simulink model "raman_updated"  (R2024b)
settings: Solver=VariableStepAuto  StartTime=0.0  StopTime=10.0  RelTol=1e-3
values from neighbouring files (symbols this model uses):
  alpha_AS_dB_km = 0.40    (= 0.4)    [Inverter_new.m]    (also in init_pv_inverter.m = 0.26)
  alpha_p_dB_km = 0.20    (= 0.2)    [Inverter_new.m]    (also in init_pv_inverter.m)
  alpha_S_dB_km = 0.20    (= 0.2)    [Inverter_new.m]    (also in init_pv_inverter.m = 0.24)
  B_rx = 1e9    (= 1000000000)    [Inverter_new.m]    (also in init_pv_inverter.m = 10000000)
  beta_AS = 1e-8    (= 1e-08)    [Inverter_new.m]    (also in init_pv_inverter.m)
  beta_S = 1e-8    (= 1e-08)    [Inverter_new.m]    (also in init_pv_inverter.m)
  delta_nu_R = c0 * raman_shift_m    [Inverter_new.m]    (also in init_pv_inverter.m = 13190868152000)
  dz_DTS = 0.5    [init_pv_inverter.m]
  I_dark = 2e-9    (= 2e-09)    [Inverter_new.m]    (also in init_pv_inverter.m = 1e-09)
  k_A = 0.7    [Inverter_new.m]
  kB = 1.380649e-23    [init_pv_inverter.m]
  M_APD = 10    [Inverter_new.m]
  N_avg = 4000    [Inverter_new.m]
  P0_laser = 70e-3    (= 0.07)    [Inverter_new.m]    (also in init_pv_inverter.m = 0.1)
  PRF = 10e3    (= 10000)    [Inverter_new.m]    (also in init_pv_inverter.m)
  q_e = 1.602176634e-19    [init_pv_inverter.m]
  R_AS = 1.0    (= 1)    [Inverter_new.m]    (also in init_pv_inverter.m = 0.9)
  R_f = 1e5    (= 100000)    [Inverter_new.m]    (also in init_pv_inverter.m)
  R_L = 1e3    (= 1000)    [Inverter_new.m]    (also in init_pv_inverter.m)
  R_S = 1.0    (= 1)    [Inverter_new.m]    (also in init_pv_inverter.m = 0.9)
  RTI = 90    [init_pv_inverter.m]
  T_ambient_fibre = Ta_K    (= 298.15)    [init_pv_inverter.m]
  T_rx = 300    [Inverter_new.m]    (also in init_pv_inverter.m = 298)
  tau_p = 2*n_g*dz_DTS/c0    [Inverter_new.m]    (also in init_pv_inverter.m = 5e-09)
  V_sat = 5    [Inverter_new.m]    (also in init_pv_inverter.m)
  x_fibre = 0:dx:L_fibre    [init_pv_inverter.m]
  x_inv_end = 7    [init_pv_inverter.m]
  x_inv_start = 5    [init_pv_inverter.m]
  z_DTS = (0:dz_DTS:L_fibre).'    [init_pv_inverter.m]
settings Model: Creator=tf  LastModifiedBy=tf

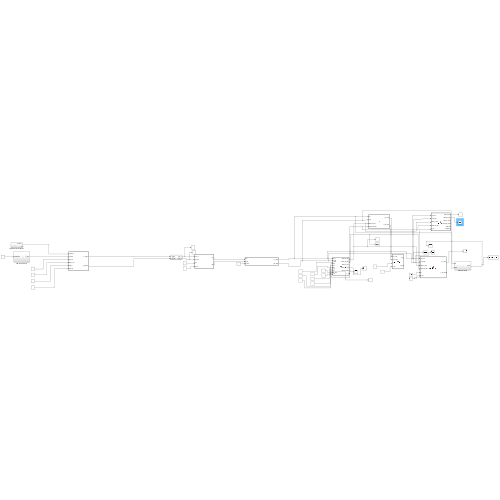
[thumbnail: Simulink's stored preview of the top-level diagram]
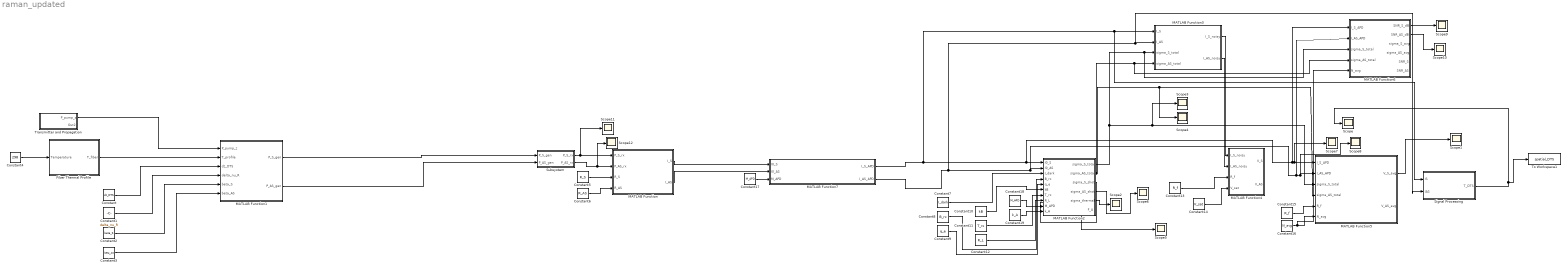
== system raman_updated ==
  Constant : Constant  Value=dz_DTS
  Constant1 : Constant  Value=delta_nu_R
  Constant10 : Constant  Value=kB
  Constant11 : Constant  Value=T_rx
  Constant12 : Constant  Value=R_L
  Constant13 : Constant  Value=R_f
  Constant14 : Constant  Value=V_sat
  Constant15 : Constant  Value=R_f
  Constant16 : Constant  Value=N_avg
  Constant17 : Constant  Value=M_APD
  Constant18 : Constant  Value=M_APD
  Constant19 : Constant  Value=k_A
  Constant2 : Constant  Value=beta_S
  Constant3 : Constant  Value=beta_AS
  Constant4 : Constant  Value=298
  Constant5 : Constant  Value=R_S
  Constant6 : Constant  Value=R_AS
  Constant7 : Constant  Value=I_dark
  Constant8 : Constant  Value=B_rx
  Constant9 : Constant  Value=q_e
  Fiber Thermal Profile : Subsystem
  MATLAB Function : MATLAB Function  TreatAsAtomicUnit=on
  MATLAB Function1 : MATLAB Function  TreatAsAtomicUnit=on
  MATLAB Function2 : MATLAB Function  TreatAsAtomicUnit=on
  MATLAB Function3 : MATLAB Function  TreatAsAtomicUnit=on
  MATLAB Function4 : MATLAB Function  TreatAsAtomicUnit=on
  MATLAB Function5 : MATLAB Function  TreatAsAtomicUnit=on
  MATLAB Function6 : MATLAB Function  TreatAsAtomicUnit=on
  MATLAB Function7 : MATLAB Function  TreatAsAtomicUnit=on
  Scope{,1..12} (13 alike) : Scope
  Signal Processing : Subsystem
  Subsystem : Subsystem
  To Workspace1 : ToWorkspace  VariableName=spatial_DTS  SaveFormat=Timeseries  SampleTime=0.01
  Transmitter and Propagation : Subsystem
  wires:
  Constant3/1 -> MATLAB Function1/6(beta_AS)
  Constant4/1 -> Fiber Thermal Profile/1(Temperature)
  Constant2/1 -> MATLAB Function1/5(beta_S)
  Fiber Thermal Profile/1(T_fiber) -> MATLAB Function1/2(T_profile)
  Constant1/1 -> MATLAB Function1/4(delta_nu_R)
  Constant/1 -> MATLAB Function1/3(dz_DTS)
  Transmitter and Propagation/1(P_pump_z) -> MATLAB Function1/1(P_pump_z)
  Subsystem/2(P_AS_rx) -> Scope12/1, MATLAB Function/2(P_AS_rx)
  Constant5/1 -> MATLAB Function/3(R_S)
  Constant6/1 -> MATLAB Function/4(R_AS)
  Constant7/1 -> MATLAB Function2/3(I_dark)
  Constant8/1 -> MATLAB Function2/4(B_rx)
  Constant9/1 -> MATLAB Function2/5(q_e)
  Constant10/1 -> MATLAB Function2/6(kB)
  Constant11/1 -> MATLAB Function2/7(T_rx)
  Constant12/1 -> MATLAB Function2/8(R_L)
  MATLAB Function2/1(sigma_S_total) -> MATLAB Function6/3(sigma_S_total), MATLAB Function3/3(sigma_S_total), Scope3/1, MATLAB Function5/3(sigma_S_total)
  Constant13/1 -> MATLAB Function4/3(R_f)
  Constant14/1 -> MATLAB Function4/4(V_sat)
  MATLAB Function2/5(sigma_thermal) -> Scope2/1
  Constant15/1 -> MATLAB Function5/5(R_f)
  Constant16/1 -> MATLAB Function6/5(N_avg), MATLAB Function5/6(N_avg)
  Signal Processing/1(T_DTS) -> Scope/1, To Workspace1/1
  MATLAB Function5/1(V_S_avg) -> Scope1/1
  MATLAB Function1/1(P_S_gen) -> Subsystem/1(P_S_gen)
  MATLAB Function1/2(P_AS_gen) -> Subsystem/2(P_AS_gen)
  Subsystem/1(P_S_rx) -> Scope11/1, MATLAB Function/1(P_S_rx)
  MATLAB Function2/3(sigma_S_shot) -> Scope5/1
  MATLAB Function/1(I_S) -> MATLAB Function7/1(I0_S)
  MATLAB Function/2(I_AS) -> MATLAB Function7/2(I0_AS)
  Constant17/1 -> MATLAB Function7/3(M_APD)
  MATLAB Function7/1(I_S_APD) -> Signal Processing/1(IS), MATLAB Function3/1(I_S), MATLAB Function6/1(I_S_APD), Scope7/1, MATLAB Function5/1(I_S_APD), MATLAB Function2/1(I0_S)
  MATLAB Function7/2(I_AS_APD) -> Signal Processing/2(IAS), MATLAB Function3/2(I_AS), MATLAB Function6/2(I_AS_APD), Scope8/1, MATLAB Function5/2(I_AS_APD), MATLAB Function2/2(I0_AS)
  Constant18/1 -> MATLAB Function2/9(M_APD)
  Constant19/1 -> MATLAB Function2/10(k_A)
  MATLAB Function3/1(I_S_noisy) -> MATLAB Function4/1(I_S_noisy)
  MATLAB Function3/2(I_AS_noisy) -> MATLAB Function4/2(I_AS_noisy)
  MATLAB Function2/4(sigma_AS_shot) -> Scope6/1
  MATLAB Function2/2(sigma_AS_total) -> MATLAB Function6/4(sigma_AS_total), MATLAB Function3/4(sigma_AS_total), Scope4/1, MATLAB Function5/4(sigma_AS_total)
  MATLAB Function6/1(SNR_S_dB) -> Scope9/1
  MATLAB Function6/2(SNR_AS_dB) -> Scope10/1

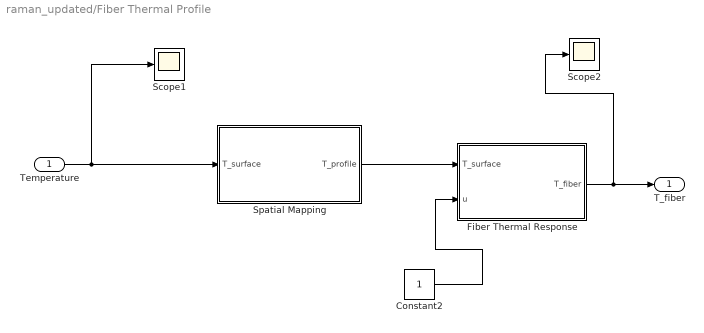
== system raman_updated/Fiber Thermal Profile ==
  Temperature : Inport
  Constant2 : Constant
  Fiber Thermal Response : Subsystem
  Scope1 : Scope
  Scope2 : Scope
  Spatial Mapping : Subsystem
  T_fiber : Outport
  wires:
  Fiber Thermal Response/1(T_fiber) -> T_fiber/1, Scope2/1
  Spatial Mapping/1(T_profile) -> Fiber Thermal Response/1(T_surface)
  Temperature/1 -> Scope1/1, Spatial Mapping/1(T_surface)
  Constant2/1 -> Fiber Thermal Response/2(u)

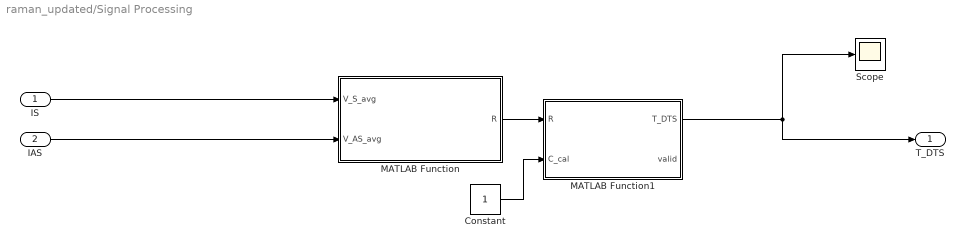
== system raman_updated/Signal Processing ==
  IS : Inport
  IAS : Inport  Port=2
  Constant : Constant
  MATLAB Function : MATLAB Function  TreatAsAtomicUnit=on
  MATLAB Function1 : MATLAB Function  TreatAsAtomicUnit=on
  Scope : Scope
  T_DTS : Outport
  wires:
  MATLAB Function/1(R) -> MATLAB Function1/1(R)
  MATLAB Function1/1(T_DTS) -> T_DTS/1, Scope/1
  IS/1 -> MATLAB Function/1(V_S_avg)
  IAS/1 -> MATLAB Function/2(V_AS_avg)
  Constant/1 -> MATLAB Function1/2(C_cal)

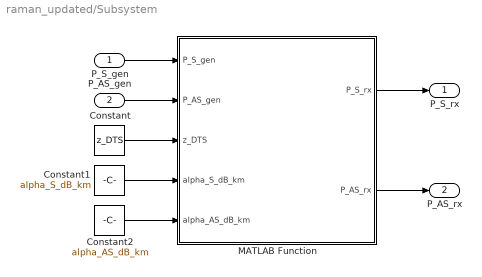
== system raman_updated/Subsystem ==
  P_S_gen : Inport
  P_AS_gen : Inport  Port=2
  Constant : Constant  Value=z_DTS
  Constant1 : Constant  Value=alpha_S_dB_km
  Constant2 : Constant  Value=alpha_AS_dB_km
  MATLAB Function : MATLAB Function  TreatAsAtomicUnit=on
  P_S_rx : Outport
  P_AS_rx : Outport  Port=2
  wires:
  P_S_gen/1 -> MATLAB Function/1(P_S_gen)
  P_AS_gen/1 -> MATLAB Function/2(P_AS_gen)
  Constant/1 -> MATLAB Function/3(z_DTS)
  Constant1/1 -> MATLAB Function/4(alpha_S_dB_km)
  Constant2/1 -> MATLAB Function/5(alpha_AS_dB_km)
  MATLAB Function/1(P_S_rx) -> P_S_rx/1
  MATLAB Function/2(P_AS_rx) -> P_AS_rx/1

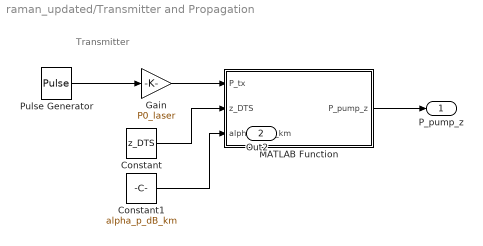
== system raman_updated/Transmitter and Propagation ==
  note: Transmitter
  Constant : Constant  Value=z_DTS
  Constant1 : Constant  Value=alpha_p_dB_km
  Gain : Gain  Gain=P0_laser
  MATLAB Function : MATLAB Function  TreatAsAtomicUnit=on
  Pulse Generator : DiscretePulseGenerator  PulseType=Time based  Period=1/PRF  PulseWidth=100*tau_p*PRF
  P_pump_z : Outport
  Out2 : Outport  Port=2
  wires:
  Constant1/1 -> MATLAB Function/3(alpha_p_dB_km)
  Pulse Generator/1 -> Gain/1
  Constant/1 -> MATLAB Function/2(z_DTS)
  Gain/1 -> MATLAB Function/1(P_tx)
  MATLAB Function/1(P_pump_z) -> P_pump_z/1

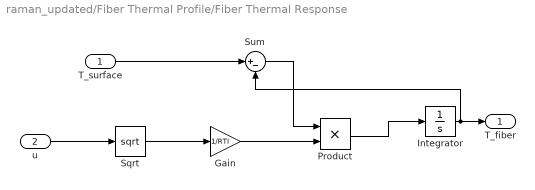
== system raman_updated/Fiber Thermal Profile/Fiber Thermal Response ==
  T_surface : Inport
  u : Inport  Port=2
  Gain : Gain  Gain=1/RTI
  Integrator : Integrator  InitialCondition=298.15
  Product : Product
  Sqrt : Sqrt
  Sum : Sum  Inputs=|+-
  T_fiber : Outport
  wires:
  u/1 -> Sqrt/1
  Gain/1 -> Product/2
  Sqrt/1 -> Gain/1
  T_surface/1 -> Sum/1
  Integrator/1 -> Sum/2, T_fiber/1
  Sum/1 -> Product/1
  Product/1 -> Integrator/1

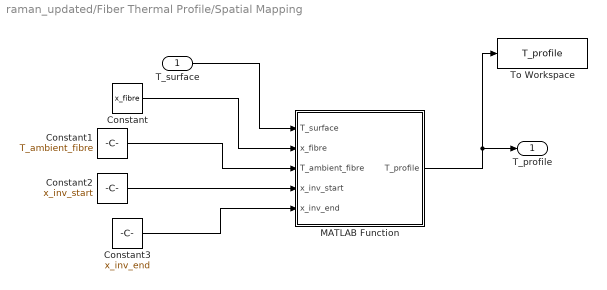
== system raman_updated/Fiber Thermal Profile/Spatial Mapping ==
  T_surface : Inport
  Constant : Constant  Value=x_fibre
  Constant1 : Constant  Value=T_ambient_fibre
  Constant2 : Constant  Value=x_inv_start
  Constant3 : Constant  Value=x_inv_end
  MATLAB Function : MATLAB Function  TreatAsAtomicUnit=on
  To Workspace : ToWorkspace  VariableName=T_profile  SampleTime=-1
      settings: Decimation=200
  T_profile : Outport
  wires:
  T_surface/1 -> MATLAB Function/1(T_surface)
  MATLAB Function/1(T_profile) -> To Workspace/1, T_profile/1
  Constant/1 -> MATLAB Function/2(x_fibre)
  Constant1/1 -> MATLAB Function/3(T_ambient_fibre)
  Constant2/1 -> MATLAB Function/4(x_inv_start)
  Constant3/1 -> MATLAB Function/5(x_inv_end)

== matlab function raman_updated/MATLAB Function4 ==
  data: I_S_noisy input; V_S output; I_AS_noisy input; R_f input; V_sat input; V_AS output
function [V_S, V_AS] = TIA_amplifier( ...
    I_S_noisy, I_AS_noisy, R_f, V_sat)

%#codegen

V_S  = R_f .* I_S_noisy;
V_AS = R_f .* I_AS_noisy;

% Saturation
V_S  = min(max(V_S,  -V_sat), V_sat);
V_AS = min(max(V_AS, -V_sat), V_sat);

end

== matlab function raman_updated/MATLAB Function5 ==
  settings: updateMethod=DISCRETE
  data: I_S_APD input; V_S_avg output; I_AS_APD input; sigma_S_total input; sigma_AS_total input; R_f input; N_avg input; V_AS_avg output
function [V_S_avg, V_AS_avg] = trace_averaging( ...
    I_S_APD, I_AS_APD, ...
    sigma_S_total, sigma_AS_total, ...
    R_f, N_avg)

%#codegen

sigma_S_avg = sigma_S_total ./ sqrt(N_avg);

sigma_AS_avg = sigma_AS_total ./ sqrt(N_avg);

nS  = randn(size(I_S_APD));
nAS = randn(size(I_AS_APD));

I_S_avg = I_S_APD + sigma_S_avg .* nS;

I_AS_avg = I_AS_APD + sigma_AS_avg .* nAS;

V_S_avg = R_f .* I_S_avg;

V_AS_avg = R_f .* I_AS_avg;

end

== matlab function raman_updated/MATLAB Function6 ==
  data: I_S_APD input; SNR_S_dB output; I_AS_APD input; sigma_S_total input; sigma_AS_total input; N_avg input; SNR_AS_dB output; sigma_S_avg output; sigma_AS_avg output; SNR_S output; SNR_AS output
function [SNR_S_dB, SNR_AS_dB, ...
          sigma_S_avg, sigma_AS_avg, ...
          SNR_S, SNR_AS] = APD_SNR( ...
          I_S_APD, I_AS_APD, ...
          sigma_S_total, sigma_AS_total, N_avg)

%#codegen

% Noise after averaging
sqrt_N = sqrt(N_avg);

sigma_S_avg  = sigma_S_total  ./ sqrt_N;
sigma_AS_avg = sigma_AS_total ./ sqrt_N;

% Linear amplitude SNR
SNR_S  = abs(I_S_APD)  ./ sigma_S_avg;
SNR_AS = abs(I_AS_APD) ./ sigma_AS_avg;

% Protect logarithm
SNR_S_safe  = max(SNR_S,  1e-12);
SNR_AS_safe = max(SNR_AS, 1e-12);

% Convert amplitude ratio to dB
SNR_S_dB  = 20 .* log10(SNR_S_safe);
SNR_AS_dB = 20 .* log10(SNR_AS_safe);

end

== matlab function raman_updated/Signal Processing/MATLAB Function ==
  data: V_S_avg input; R output; V_AS_avg input
function R = RamanRatio(V_S_avg, V_AS_avg)

%#codegen

eps_sig = 1e-15;

VS  = max(V_S_avg,  eps_sig);
VAS = max(V_AS_avg, eps_sig);

R = VAS ./ VS;

end

== matlab function raman_updated/Signal Processing/MATLAB Function1 ==
  data: R input; T_DTS output; C_cal input; valid output
function [T_DTS, valid] = Reconstruct_Temperature(R, C_cal)

%#codegen

h  = 6.62607015e-34;
c0 = 2.99792458e8;
kB = 1.380649e-23;

raman_shift_cm = 440;
raman_shift_m  = raman_shift_cm * 100;

Theta_R = h*c0*raman_shift_m/kB;

R_corr = R ./ C_cal;

T_DTS = NaN(size(R_corr));
valid = false(size(R_corr));

for i = 1:numel(R_corr)

    % Physical range required by this ratio convention
    if R_corr(i) > 0 && R_corr(i) < 1

        T_DTS(i) = ...
            -Theta_R / log(R_corr(i));

        valid(i) = true;

    end
end

end

== matlab function raman_updated/MATLAB Function7 ==
  data: I0_S input; I_S_APD output; I0_AS input; M_APD input; I_AS_APD output
function [I_S_APD, I_AS_APD] = APD_gain( ...
    I0_S, I0_AS, M_APD)

%#codegen

I_S_APD  = M_APD .* I0_S;
I_AS_APD = M_APD .* I0_AS;



end

== matlab function raman_updated/MATLAB Function1 ==
  data: P_pump_z input; P_S_gen output; T_profile input; dz_DTS input; delta_nu_R input; beta_S input; beta_AS input; P_AS_gen output
function [P_S_gen, P_AS_gen] = RamanScatterer( ...
    P_pump_z, T_profile, dz_DTS, delta_nu_R, beta_S, beta_AS)

% Physical constants
h  = 6.62607015e-34;      % Planck constant [J s]
kB = 1.380649e-23;        % Boltzmann constant [J/K]

% Force spatial vectors into columns
P_pump_z = P_pump_z(:);
T_profile = T_profile(:);

% Raman phonon occupation number
x = h * delta_nu_R ./ (kB .* T_profile);

n_R = 1 ./ (exp(x) - 1);

% Locally generated spontaneous Raman backscatter power
P_AS_gen = P_pump_z .* beta_AS .* n_R .* dz_DTS;

P_S_gen = P_pump_z .* beta_S .* (n_R + 1) .* dz_DTS;

end

== matlab function raman_updated/Subsystem/MATLAB Function ==
  data: P_S_gen input; P_S_rx output; P_AS_gen input; z_DTS input; alpha_S_dB_km input; alpha_AS_dB_km input; P_AS_rx output
function [P_S_rx, P_AS_rx] = RamanReturnPropagation( ...
    P_S_gen, P_AS_gen, z_DTS, alpha_S_dB_km, alpha_AS_dB_km)

% Force spatial vectors to columns
P_S_gen  = P_S_gen(:);
P_AS_gen = P_AS_gen(:);
z_DTS    = z_DTS(:);

% Return-path transmission from position z back to receiver at z = 0
H_S = 10.^(-alpha_S_dB_km .* z_DTS ./ 10000);
H_AS = 10.^(-alpha_AS_dB_km .* z_DTS ./ 10000);

% Raman powers arriving at receiver
P_S_rx = P_S_gen .* H_S;
P_AS_rx = P_AS_gen .* H_AS;

end

== matlab function raman_updated/Transmitter and Propagation/MATLAB Function ==
  data: P_tx input; P_pump_z output; z_DTS input; alpha_p_dB_km input
function P_pump_z = pump_propagation( ...
    P_tx, z_DTS, alpha_p_dB_km)

% Forward propagation of pump optical power.
%
% P_tx          : launched optical power [W]
% z_DTS         : fibre position vector [m]
% alpha_p_dB_km : pump attenuation [dB/km]
%
% P_pump_z      : pump power at each fibre position [W]

P_pump_z = P_tx .* ...
    10.^(-alpha_p_dB_km .* z_DTS ./ 10000);

end

== matlab function raman_updated/Fiber Thermal Profile/Spatial Mapping/MATLAB Function ==
  data: T_surface input; T_profile output; x_fibre input; T_ambient_fibre input; x_inv_start input; x_inv_end input
function T_profile = spatial_mapping(T_surface, x_fibre, ...
    T_ambient_fibre, x_inv_start, x_inv_end)
%#codegen

N = 41;

% Fixed-size output
T_profile = T_ambient_fibre .* ones(1,N);

% Inverter sensing region
idx = (x_fibre >= x_inv_start) & ...
      (x_fibre <= x_inv_end);

% Apply inverter surface temperature
T_profile(idx) = T_surface;

end

== matlab function raman_updated/MATLAB Function ==
  data: P_S_rx input; I_S output; P_AS_rx input; R_S input; R_AS input; I_AS output
function [I_S, I_AS] = photodetector(P_S_rx, P_AS_rx, R_S, R_AS)

I_S  = R_S  .* P_S_rx;
I_AS = R_AS .* P_AS_rx;

end

== matlab function raman_updated/MATLAB Function2 ==
  data: I0_S input; sigma_S_total output; I0_AS input; I_dark input; B_rx input; q_e input; sigma_AS_total output; kB input; T_rx input; R_L input; sigma_S_shot output; sigma_AS_shot output; sigma_thermal output; M_APD input; k_A input; F_A output
function [sigma_S_total, sigma_AS_total, ...
          sigma_S_shot, sigma_AS_shot, ...
          sigma_thermal, F_A] = receiver_noise_APD( ...
          I0_S, I0_AS, I_dark, B_rx, q_e, ...
          kB, T_rx, R_L, M_APD, k_A)

%#codegen

% APD excess noise factor
F_A = k_A .* M_APD + ...
      (1-k_A) .* (2 - 1./M_APD);

% APD shot noise
sigma_S_shot = sqrt( ...
    2*q_e .* B_rx .* M_APD.^2 .* F_A .* ...
    (I0_S + I_dark));

sigma_AS_shot = sqrt( ...
    2*q_e .* B_rx .* M_APD.^2 .* F_A .* ...
    (I0_AS + I_dark));

% Receiver thermal noise
sigma_thermal = sqrt( ...
    4*kB*T_rx*B_rx/R_L);

% Total receiver noise
sigma_S_total = sqrt( ...
    sigma_S_shot.^2 + sigma_thermal.^2);

sigma_AS_total = sqrt( ...
    sigma_AS_shot.^2 + sigma_thermal.^2);


end

== matlab function raman_updated/MATLAB Function3 ==
  settings: updateMethod=DISCRETE
  data: I_S input; I_S_noisy output; I_AS input; sigma_S_total input; sigma_AS_total input; I_AS_noisy output
function [I_S_noisy, I_AS_noisy] = inject_noise( ...
    I_S, I_AS, sigma_S_total, sigma_AS_total)

%#codegen

nS  = randn(size(I_S));
nAS = randn(size(I_AS));

I_S_noisy  = I_S  + sigma_S_total  .* nS;
I_AS_noisy = I_AS + sigma_AS_total .* nAS;

end
